simulink model "LQR_controller"  (R2017a)
settings: Solver=VariableStepAuto  StartTime=0.0  StopTime=10.0  RelTol=1e-3
settings Model: Creator=lngemesce  LastModifiedBy=lngemesce

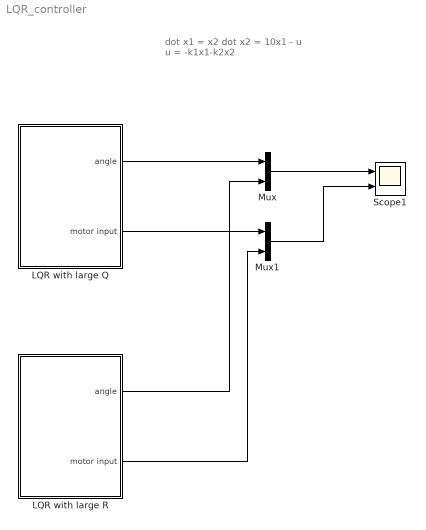
== system LQR_controller ==
  note: dot x1 = x2
      | dot x2 = 10x1 - u
      | u = -k1x1-k2x2
  LQR with large Q : Subsystem
  "LQR with large R " : Subsystem
  Mux : Mux  Inputs=2
  Mux1 : Mux  Inputs=2
  Scope1 : Scope  NumInputPorts=2
  wires:
  LQR with large Q/1(angle) -> Mux/1
  "LQR with large R "/1(angle) -> Mux/2
  Mux/1 -> Scope1/1
  LQR with large Q/2(motor input) -> Mux1/1
  "LQR with large R "/2(motor input) -> Mux1/2
  Mux1/1 -> Scope1/2

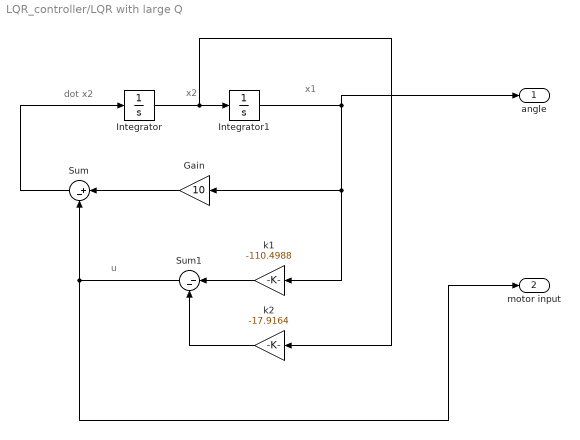
== system LQR_controller/LQR with large Q ==
  note: u
  note: x1
  note: x2
  note: dot x2
  Gain : Gain  Gain=10
  Integrator : Integrator
  Integrator1 : Integrator  InitialCondition=30/180*pi
  Sum : Sum  Inputs=|+-
  Sum1 : Sum  Inputs=|--
  k1 : Gain  Gain=-110.4988
  k2 : Gain  Gain=-17.9164
  angle : Outport
  motor input : Outport  Port=2
  wires:
  k1/1 -> Sum1/1
  Gain/1 -> Sum/1
  k2/1 -> Sum1/2
  Sum1/1 -> motor input/1, Sum/2
  Integrator1/1 -> angle/1, k1/1, Gain/1
  Integrator/1 -> k2/1, Integrator1/1
  Sum/1 -> Integrator/1

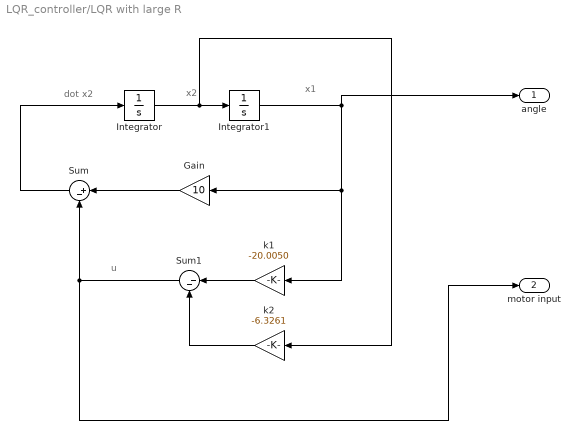
== system LQR_controller/LQR with large R  ==
  note: dot x2
  note: x2
  note: x1
  note: u
  Gain : Gain  Gain=10
  Integrator : Integrator
  Integrator1 : Integrator  InitialCondition=30/180*pi
  Sum : Sum  Inputs=|+-
  Sum1 : Sum  Inputs=|--
  k1 : Gain  Gain=-20.0050
  k2 : Gain  Gain=-6.3261
  angle : Outport
  motor input : Outport  Port=2
  wires:
  Sum/1 -> Integrator/1
  Integrator/1 -> Integrator1/1, k2/1
  Integrator1/1 -> Gain/1, k1/1, angle/1
  Sum1/1 -> Sum/2, motor input/1
  k2/1 -> Sum1/2
  Gain/1 -> Sum/1
  k1/1 -> Sum1/1
